simulink model "draft3"  (R2024b)
settings: Solver=VariableStepAuto  StartTime=0.0  StopTime=10  RelTol=1e-3  AbsTol=1e-3
settings Model: Creator=sakhs  LastModifiedBy=sakhs
settings SolverCC: AutoScaleAbsTol=off  AlgebraicLoopSolver=TrustRegion  MaxZcPerStep=1
settings DebuggingCC: UnconnectedInputMsg=warning  UnconnectedOutputMsg=warning  UnconnectedLineMsg=warning  SymbolicDimsDataTypeCodeGenerationDiagnostic=none
settings ModelReferenceCC: EnableRefExpFcnMdlSchedulingChecks=on
settings SFSimCC: CustomCodeUndefinedFunction=UseInterfaceOnly
settings RTWCC: GPUComputeCapability=3.5  DLArmComputeVersion=19.05
settings SimscapeCC: SimscapeLogType=all  SimscapeLogSimulationStatistics=on  SimscapeLogDataHistory=10000

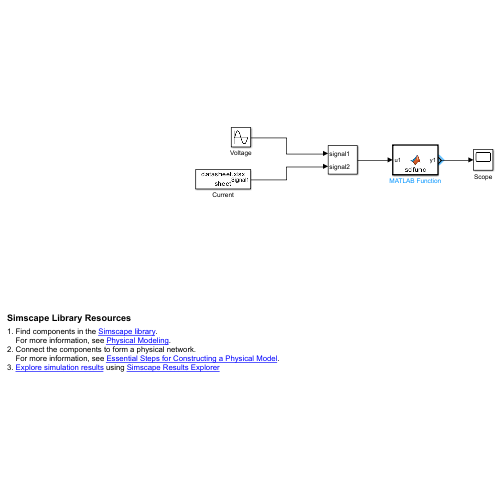
[thumbnail: Simulink's stored preview of the top-level diagram]
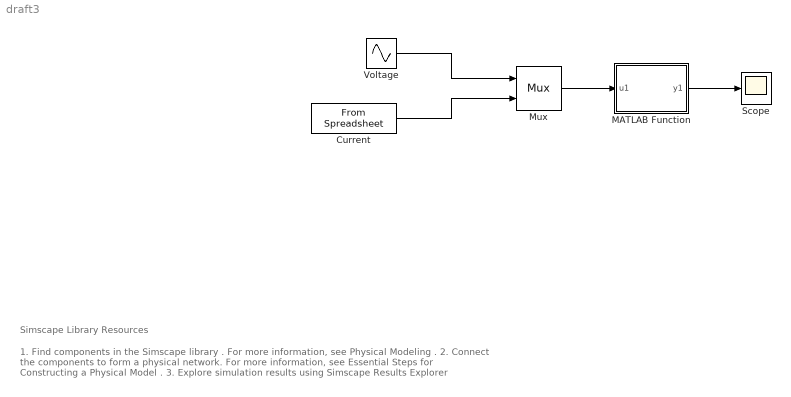
== system draft3 ==
  note: 1. Find components in the Simscape library .
      | For more information, see Physical Modeling .
      | 2. Connect the components to form a physical network.
      | For more information, see Essential Steps for Constructing a Physical Model .
      | 3. Explore simulation results using Simscape Results Explorer
  note: Simscape Library Resources
  Current : FromSpreadsheet  FileName=datasheet.xlsx  SheetName=sheet  Range=T2:U100  SampleTime=1
  MATLAB Function : MATLAB Function  TreatAsAtomicUnit=on
  Mux : Mux  Inputs=2
      settings: DisplayOption=signals
  Scope : Scope
  Voltage : Sin  Amplitude=220*1.414  Frequency=50  SampleTime=0
  wires:
  Voltage/1 -> Mux/1
  Current/1 -> Mux/2
  Mux/1 -> MATLAB Function/1(u1)
  MATLAB Function/1(y1) -> Scope/1

== matlab function draft3/MATLAB Function ==
  data: u1 input; y1 output
function y1 = scifunc(u1)
    if abs(u1(1)) > 220 && u1(2) == 1
        y1 = 1; % Tampering confirmed
    else
        y1 = 0; % Normal
    end
end
